simulink model "Tradespace"  (R2017a)
settings: Solver=VariableStepAuto  StartTime=0.0  StopTime=10.0  RelTol=1e-3
settings Model: Creator=romain  LastModifiedBy=romain

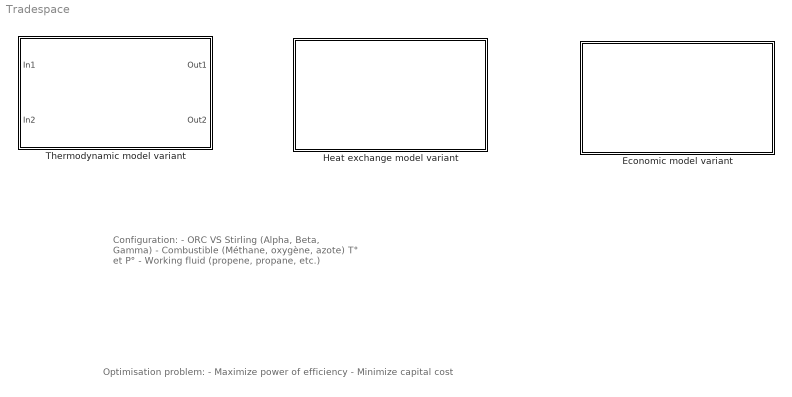
== system Tradespace ==
  note: Configuration:
      |
      | - ORC VS Stirling (Alpha, Beta, Gamma)
      | - Combustible (Méthane, oxygène, azote) T° et P°
      | - Working fluid (propene, propane, etc.)
  note: Optimisation problem:
      |
      | - Maximize power of efficiency
      | - Minimize capital cost
  Economic model variant : Subsystem  Variant=on  VariantControl=Variant1  OverrideUsingVariant=Variant1
  Heat exchange model variant : Subsystem  Variant=on  VariantControl=Variant1  OverrideUsingVariant=Variant1
  Thermodynamic model variant : Subsystem  Variant=on  VariantControl=Variant1  OverrideUsingVariant=Variant1

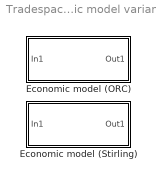
== system Tradespace/Economic model variant ==
  Economic model (ORC) : Subsystem  VariantControl=Variant
  Economic model (Stirling) : Subsystem  VariantControl=Variant1

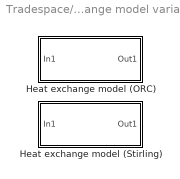
== system Tradespace/Heat exchange model variant ==
  Heat exchange model (ORC) : Subsystem  VariantControl=Variant
  Heat exchange model (Stirling) : Subsystem  VariantControl=Variant1

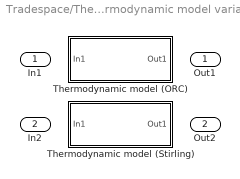
== system Tradespace/Thermodynamic model variant ==
  In1 : Inport
  In2 : Inport  Port=2
  Thermodynamic model (ORC) : Subsystem  VariantControl=Variant
  Thermodynamic model (Stirling) : Subsystem  VariantControl=Variant1
  Out1 : Outport
  Out2 : Outport  Port=2

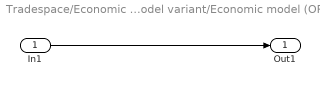
== system Tradespace/Economic model variant/Economic model (ORC) ==
  In1 : Inport
  Out1 : Outport
  wires:
  In1/1 -> Out1/1

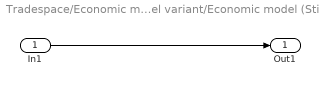
== system Tradespace/Economic model variant/Economic model (Stirling) ==
  In1 : Inport
  Out1 : Outport
  wires:
  In1/1 -> Out1/1

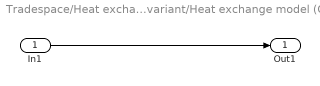
== system Tradespace/Heat exchange model variant/Heat exchange model (ORC) ==
  In1 : Inport
  Out1 : Outport
  wires:
  In1/1 -> Out1/1

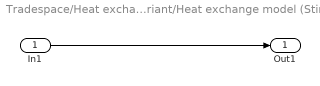
== system Tradespace/Heat exchange model variant/Heat exchange model (Stirling) ==
  In1 : Inport
  Out1 : Outport
  wires:
  In1/1 -> Out1/1

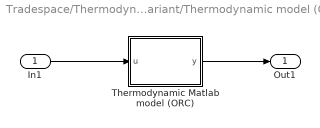
== system Tradespace/Thermodynamic model variant/Thermodynamic model (ORC) ==
  In1 : Inport
  Thermodynamic Matlab model (ORC) : MATLAB Function  TreatAsAtomicUnit=on
  Out1 : Outport
  wires:
  In1/1 -> Thermodynamic Matlab model (ORC)/1(u)
  Thermodynamic Matlab model (ORC)/1(y) -> Out1/1

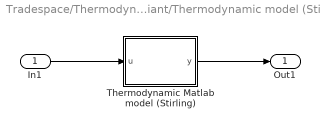
== system Tradespace/Thermodynamic model variant/Thermodynamic model (Stirling) ==
  In1 : Inport
  Thermodynamic Matlab model (Stirling) : MATLAB Function  TreatAsAtomicUnit=on
  Out1 : Outport
  wires:
  In1/1 -> Thermodynamic Matlab model (Stirling)/1(u)
  Thermodynamic Matlab model (Stirling)/1(y) -> Out1/1

== matlab function Tradespace/Thermodynamic model variant/Thermodynamic model (Stirling)/Thermodynamic Matlab model (Stirling) ==
  data: u input; y output
function y = fcn(u)

y = u;

== matlab function Tradespace/Thermodynamic model variant/Thermodynamic model (ORC)/Thermodynamic Matlab model (ORC) ==
  data: u input; y output
function y = fcn(u)

y = u;
